simulink model "plant"  (R2017a)
settings: Solver=FixedStepAuto  StartTime=0.0  StopTime=2  FixedStep=0.0002  RelTol=1e-3
settings Model: Creator=saturn  LastModifiedBy=saturn

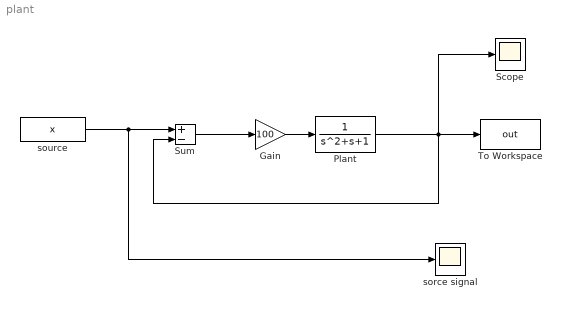
== system plant ==
  Gain : Gain  Gain=100
  Plant : TransferFcn  Denominator=[1 1 1]
  Scope : Scope
  Sum : Sum  Inputs=+-
  To Workspace : ToWorkspace  VariableName=out  SampleTime=-1
      settings: Save2DSignal=2-D array (concatenate along first dimension)
  sorce signal : Scope
  "source " : FromWorkspace  VariableName=x  SampleTime=0  OutputAfterFinalValue=Setting to zero
  wires:
  Plant/1 -> Sum/2, Scope/1, To Workspace/1
  "source "/1 -> sorce signal/1, Sum/1
  Sum/1 -> Gain/1
  Gain/1 -> Plant/1
